simulink model "calculateDutyCycle"  (R2022b)
settings: Solver=VariableStepAuto  StartTime=0.0  StopTime=10.0  RelTol=1e-3
settings Model: Creator=pc  LastModifiedBy=pc

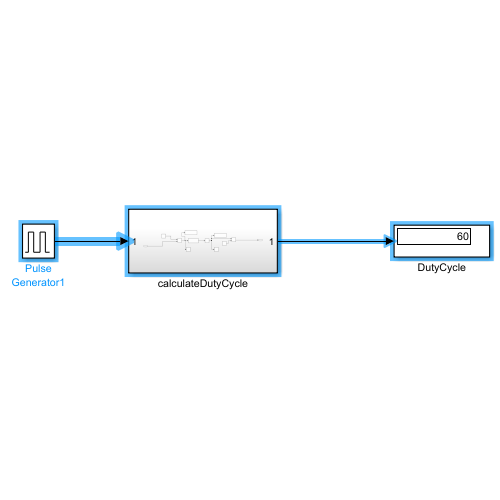
[thumbnail: Simulink's stored preview of the top-level diagram]
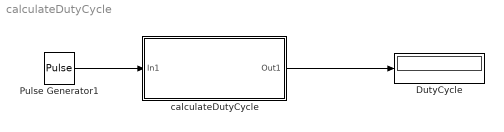
== system calculateDutyCycle ==
  DutyCycle : Display
  Pulse Generator1 : DiscretePulseGenerator  PulseType=Time based  Amplitude=5  Period=10  PulseWidth=60
  calculateDutyCycle : Subsystem
  wires:
  calculateDutyCycle/1(Out1) -> DutyCycle/1
  Pulse Generator1/1 -> calculateDutyCycle/1(In1)

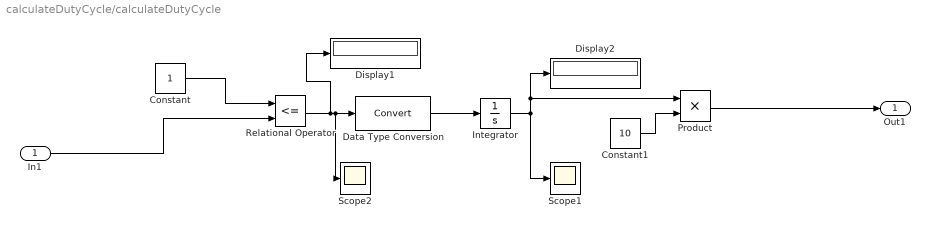
== system calculateDutyCycle/calculateDutyCycle ==
  In1 : Inport
  Constant : Constant
  Constant1 : Constant  Value=10
  Data Type Conversion : DataTypeConversion  SaturateOnIntegerOverflow=off  RndMeth=Floor
  Display1 : Display
  Display2 : Display
  Integrator : Integrator
  Product : Product
  Relational Operator : RelationalOperator  Operator=<=  OutDataTypeStr=boolean  RndMeth=Simplest  InputSameDT=off
  Scope1 : Scope
  Scope2 : Scope
  Out1 : Outport
  wires:
  Integrator/1 -> Product/1, Display2/1, Scope1/1
  Constant/1 -> Relational Operator/1
  Relational Operator/1 -> Display1/1, Scope2/1, Data Type Conversion/1
  Data Type Conversion/1 -> Integrator/1
  In1/1 -> Relational Operator/2
  Constant1/1 -> Product/2
  Product/1 -> Out1/1
